simulink model "pmsm_vector_ctrl_osm_2021_07_20"  (R2020a)
settings: Solver=daessc  StartTime=0.0  StopTime=simlength  MaxStep=Ts/10
values from neighbouring files (symbols this model uses):
  dead_time = 0    [init_pmsm_2021_07_20_newDesign.m]    (also in init_pmsm_2021_07_20_oldDesign.m)
  delayINV_modA = 0    [init_pmsm_2021_07_20_newDesign.m]    (also in init_pmsm_2021_07_20_oldDesign.m)
  fPWM_INV = 8e3    (= 8000)    [init_pmsm_2021_07_20_newDesign.m]    (also in init_pmsm_2021_07_20_oldDesign.m)
  Ibez = 550    [init_pmsm_2021_07_20_newDesign.m]    (also in init_pmsm_2021_07_20_oldDesign.m)
  Jm = 1    [init_pmsm_2021_07_20_newDesign.m]    (also in init_pmsm_2021_07_20_oldDesign.m)
  ki = 18    [init_pmsm_2021_07_20_newDesign.m]    (also in init_pmsm_2021_07_20_oldDesign.m)
  kp = 2    [init_pmsm_2021_07_20_newDesign.m]    (also in init_pmsm_2021_07_20_oldDesign.m)
  Ld = 2.77e-3    (= 0.00277)    [init_pmsm_2021_07_20_newDesign.m]    (also in init_pmsm_2021_07_20_oldDesign.m = 0.00267)
  Lq = 3.77e-3    (= 0.00377)    [init_pmsm_2021_07_20_newDesign.m]    (also in init_pmsm_2021_07_20_oldDesign.m = 0.00328)
  number_poles = 8    [init_pmsm_2021_07_20_newDesign.m]    (also in init_pmsm_2021_07_20_oldDesign.m)
  psi_m = 0.5    [init_pmsm_2021_07_20_newDesign.m]    (also in init_pmsm_2021_07_20_oldDesign.m = 0.37)
  simlength = 5    [init_pmsm_2021_07_20_newDesign.m]    (also in init_pmsm_2021_07_20_oldDesign.m)
  Tc = 1e-5    (= 1e-05)    [init_pmsm_2021_07_20_newDesign.m]    (also in init_pmsm_2021_07_20_oldDesign.m)
  Ts = tPWM_INV/2    (= 3.125e-05)    [init_pmsm_2021_07_20_newDesign.m]    (also in init_pmsm_2021_07_20_oldDesign.m)
libraries: nesl_utility x25, fl_lib x23, ee_lib x6, flexshaft_lib x1, pmsm_uvw_lib x1
(part 2 of 2)

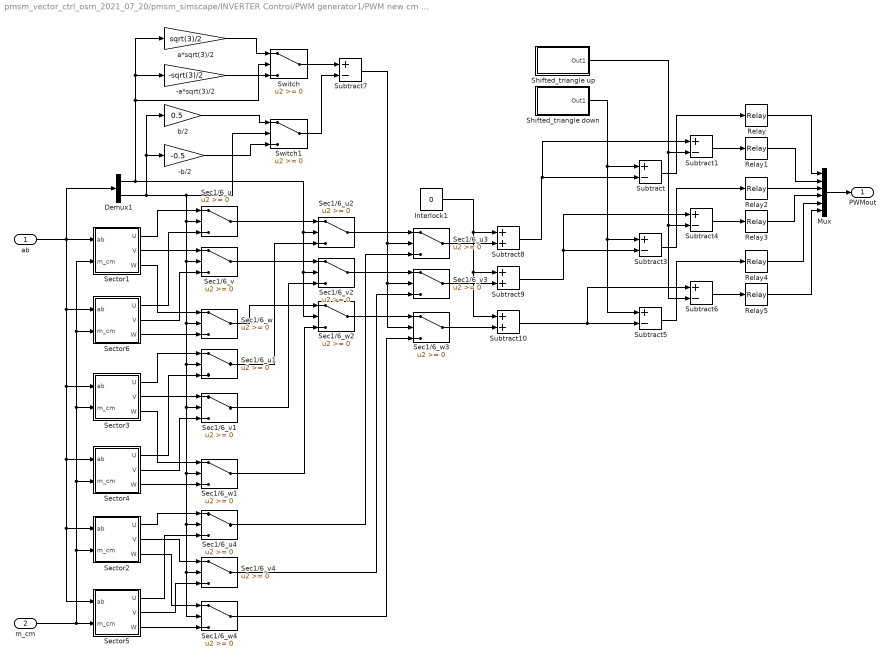
== system pmsm_vector_ctrl_osm_2021_07_20/pmsm_simscape/INVERTER Control/PWM generator1/PWM new cm modulation ==
  ab : Inport
  m_cm : Inport  Port=2
  -a*sqrt(3)/2 : Gain  Gain=-sqrt(3)/2
  -b/2 : Gain  Gain=-0.5
  Demux1 : Demux  Outputs=2
  Interlock1 : Constant  Value=0
  Mux : Mux  Inputs=6
  Relay{,1..5} (6 alike) : Relay  OnOutputValue=15
  Sec1/6_u{,1..4} (5 alike) : Switch
  Sec1/6_v{,1..4} (5 alike) : Switch
  Sec1/6_w{,1..4} (5 alike) : Switch
  Sector1 : Subsystem
  Sector2 : Subsystem
  Sector3 : Subsystem
  Sector4 : Subsystem
  Sector5 : Subsystem
  Sector6 : Subsystem
  Shifted_triangle down : Subsystem
  Shifted_triangle up : Subsystem
  Subtract{,1,3..7} (7 alike) : Sum  Inputs=+-
  Subtract10 : Sum
  Subtract8 : Sum
  Subtract9 : Sum
  Switch : Switch
  Switch1 : Switch
  a*sqrt(3)/2 : Gain  Gain=sqrt(3)/2
  b/2 : Gain  Gain=0.5
  PWMout : Outport
  wires:
  m_cm/1 -> Sector5/2(m_cm), Sector4/2(m_cm), Sector3/2(m_cm), Sector6/2(m_cm), Sector1/2(m_cm), Sector2/2(m_cm)
  Sector5/3(W) -> Sec1/6_w4/3
  Sector5/2(V) -> Sec1/6_v4/3
  Sector5/1(U) -> Sec1/6_u4/3
  Sector2/3(W) -> Sec1/6_w4/1
  Sector2/2(V) -> Sec1/6_v4/1
  Sector2/1(U) -> Sec1/6_u4/1
  Sec1/6_w4/1 -> Sec1/6_w3/3
  Sec1/6_v4/1 -> Sec1/6_v3/3
  Sec1/6_u4/1 -> Sec1/6_u3/3
  Subtract7/1 -> Sec1/6_u3/2, Sec1/6_v3/2, Sec1/6_w3/2
  Sec1/6_w2/1 -> Sec1/6_w3/1
  Sec1/6_v2/1 -> Sec1/6_v3/1
  Sec1/6_u2/1 -> Sec1/6_u3/1
  Demux1/1 -> Sec1/6_w2/2, Sec1/6_v2/2, Sec1/6_u2/2, a*sqrt(3)/2/1, -a*sqrt(3)/2/1, Switch/2
  Sector4/3(W) -> Sec1/6_w1/3
  Sector4/2(V) -> Sec1/6_v1/3
  Sector4/1(U) -> Sec1/6_u1/3
  Sector3/3(W) -> Sec1/6_w1/1
  Sector3/2(V) -> Sec1/6_v1/1
  Sector3/1(U) -> Sec1/6_u1/1
  Sec1/6_w1/1 -> Sec1/6_w2/3
  Sec1/6_v1/1 -> Sec1/6_v2/3
  Sec1/6_u1/1 -> Sec1/6_u2/3
  Sec1/6_w/1 -> Sec1/6_w2/1
  Sec1/6_v/1 -> Sec1/6_v2/1
  Sec1/6_u/1 -> Sec1/6_u2/1
  Demux1/2 -> Switch1/2, Sec1/6_w4/2, Sec1/6_v4/2, Sec1/6_u4/2, Sec1/6_w1/2, Sec1/6_v1/2, Sec1/6_u1/2, Sec1/6_w/2, Sec1/6_v/2, Sec1/6_u/2, -b/2/1, b/2/1
  Sector6/3(W) -> Sec1/6_w/3
  Sector6/2(V) -> Sec1/6_v/3
  Sector6/1(U) -> Sec1/6_u/3
  Sector1/3(W) -> Sec1/6_w/1
  Sector1/2(V) -> Sec1/6_v/1
  Sector1/1(U) -> Sec1/6_u/1
  Switch1/1 -> Subtract7/2
  Switch/1 -> Subtract7/1
  a*sqrt(3)/2/1 -> Switch/1
  -a*sqrt(3)/2/1 -> Switch/3
  -b/2/1 -> Switch1/3
  b/2/1 -> Switch1/1
  ab/1 -> Demux1/1, Sector1/1(ab), Sector6/1(ab), Sector3/1(ab), Sector4/1(ab), Sector2/1(ab), Sector5/1(ab)
  Subtract6/1 -> Relay5/1
  Subtract5/1 -> Relay4/1
  Subtract4/1 -> Relay3/1
  Subtract3/1 -> Relay2/1
  Shifted_triangle up/1(Out1) -> Subtract6/2, Subtract4/2, Subtract1/2
  Subtract1/1 -> Relay1/1
  Subtract/1 -> Relay/1
  Shifted_triangle down/1(Out1) -> Subtract5/1, Subtract3/1, Subtract/1
  Mux/1 -> PWMout/1
  Relay/1 -> Mux/1
  Relay1/1 -> Mux/2
  Relay2/1 -> Mux/3
  Relay3/1 -> Mux/4
  Relay4/1 -> Mux/5
  Relay5/1 -> Mux/6
  Sec1/6_u3/1 -> Subtract8/2
  Sec1/6_v3/1 -> Subtract9/2
  Sec1/6_w3/1 -> Subtract10/2
  Subtract10/1 -> Subtract6/1, Subtract5/2
  Subtract9/1 -> Subtract4/1, Subtract3/2
  Subtract8/1 -> Subtract1/1, Subtract/2
  Interlock1/1 -> Subtract8/1, Subtract9/1, Subtract10/1

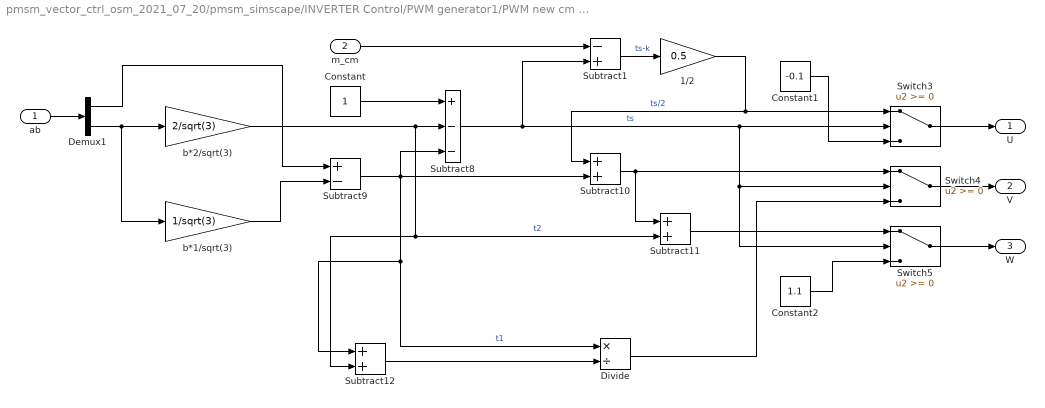
== system pmsm_vector_ctrl_osm_2021_07_20/pmsm_simscape/INVERTER Control/PWM generator1/PWM new cm modulation/Sector1 ==
  ab : Inport
  m_cm : Inport  Port=2
  1/2 : Gain  Gain=0.5
  Constant : Constant
  Constant1 : Constant  Value=-0.1
  Constant2 : Constant  Value=1.1
  Demux1 : Demux  Outputs=2
  Divide : Product  Inputs=*/
  Subtract1 : Sum  Inputs=-+
  Subtract10 : Sum
  Subtract11 : Sum
  Subtract12 : Sum
  Subtract8 : Sum  Inputs=+--
  Subtract9 : Sum  Inputs=+-
  Switch3 : Switch
  Switch4 : Switch
  Switch5 : Switch
  b*1/sqrt(3) : Gain  Gain=1/sqrt(3)
  b*2/sqrt(3) : Gain  Gain=2/sqrt(3)
  U : Outport
  V : Outport  Port=2
  W : Outport  Port=3
  wires:
  m_cm/1 -> Subtract1/1
  Switch5/1 -> W/1
  Switch4/1 -> V/1
  Switch3/1 -> U/1
  ab/1 -> Demux1/1
  Subtract8/1 -> Switch4/2, Switch5/2, Switch3/2, Subtract1/2  "ts"
  Constant/1 -> Subtract8/1
  b*2/sqrt(3)/1 -> Subtract8/2, Subtract12/2, Subtract11/2  "t2"
  Subtract9/1 -> Subtract12/1, Divide/1, Subtract10/2, Subtract8/3  "t1"
  b*1/sqrt(3)/1 -> Subtract9/2
  Subtract1/1 -> 1/2/1  "ts-k"
  Subtract10/1 -> Subtract11/1, Switch4/1
  Subtract11/1 -> Switch5/1
  Constant1/1 -> Switch3/3
  Subtract12/1 -> Divide/2
  Constant2/1 -> Switch5/3
  Divide/1 -> Switch4/3
  Demux1/1 -> Subtract9/1
  Demux1/2 -> b*2/sqrt(3)/1, b*1/sqrt(3)/1
  1/2/1 -> Switch3/1, Subtract10/1  "ts/2"

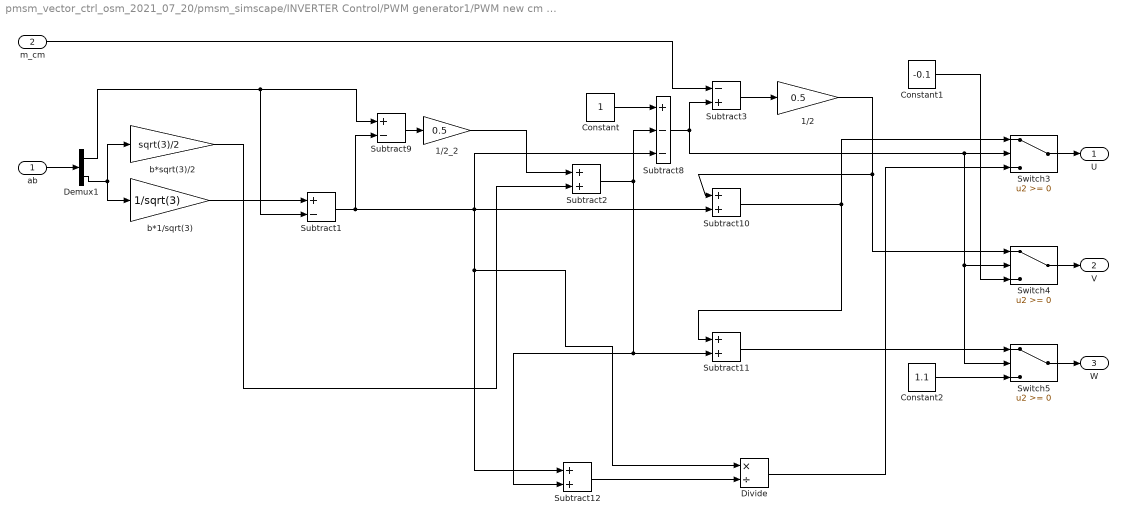
== system pmsm_vector_ctrl_osm_2021_07_20/pmsm_simscape/INVERTER Control/PWM generator1/PWM new cm modulation/Sector2 ==
  ab : Inport
  m_cm : Inport  Port=2
  1/2 : Gain  Gain=0.5
  1/2_2 : Gain  Gain=0.5
  Constant : Constant
  Constant1 : Constant  Value=-0.1
  Constant2 : Constant  Value=1.1
  Demux1 : Demux  Outputs=2
  Divide : Product  Inputs=*/
  Subtract1 : Sum  Inputs=+-
  Subtract{2,10..12} (4 alike) : Sum
  Subtract3 : Sum  Inputs=-+
  Subtract8 : Sum  Inputs=+--
  Subtract9 : Sum  Inputs=+-
  Switch3 : Switch
  Switch4 : Switch
  Switch5 : Switch
  b*1/sqrt(3) : Gain  Gain=1/sqrt(3)
  b*sqrt(3)/2 : Gain  Gain=sqrt(3)/2
  U : Outport
  V : Outport  Port=2
  W : Outport  Port=3
  wires:
  1/2/1 -> Switch4/1, Subtract10/1
  m_cm/1 -> Subtract3/1
  Subtract10/1 -> Subtract11/1, Switch3/1
  Constant2/1 -> Switch5/3
  Divide/1 -> Switch3/3
  Constant1/1 -> Switch4/3
  Subtract3/1 -> 1/2/1
  Subtract2/1 -> Subtract11/2, Subtract12/2, Subtract8/2
  b*sqrt(3)/2/1 -> Subtract2/2
  1/2_2/1 -> Subtract2/1
  Subtract9/1 -> 1/2_2/1
  Subtract1/1 -> Subtract9/2, Subtract8/3, Subtract10/2, Divide/1, Subtract12/1
  b*1/sqrt(3)/1 -> Subtract1/1
  Switch5/1 -> W/1
  Switch4/1 -> V/1
  Switch3/1 -> U/1
  ab/1 -> Demux1/1
  Subtract8/1 -> Switch5/2, Switch4/2, Switch3/2, Subtract3/2
  Constant/1 -> Subtract8/1
  Subtract11/1 -> Switch5/1
  Subtract12/1 -> Divide/2
  Demux1/1 -> Subtract1/2, Subtract9/1
  Demux1/2 -> b*sqrt(3)/2/1, b*1/sqrt(3)/1

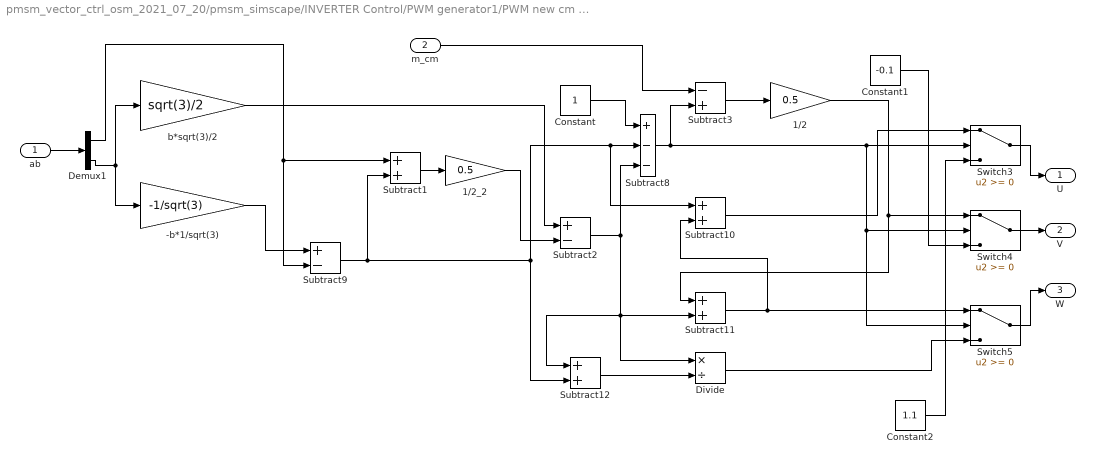
== system pmsm_vector_ctrl_osm_2021_07_20/pmsm_simscape/INVERTER Control/PWM generator1/PWM new cm modulation/Sector3 ==
  ab : Inport
  m_cm : Inport  Port=2
  -b*1/sqrt(3) : Gain  Gain=-1/sqrt(3)
  1/2 : Gain  Gain=0.5
  1/2_2 : Gain  Gain=0.5
  Constant : Constant
  Constant1 : Constant  Value=-0.1
  Constant2 : Constant  Value=1.1
  Demux1 : Demux  Outputs=2
  Divide : Product  Inputs=*/
  Subtract{1,10..12} (4 alike) : Sum
  Subtract2 : Sum  Inputs=+-
  Subtract3 : Sum  Inputs=-+
  Subtract8 : Sum  Inputs=+--
  Subtract9 : Sum  Inputs=+-
  Switch3 : Switch
  Switch4 : Switch
  Switch5 : Switch
  b*sqrt(3)/2 : Gain  Gain=sqrt(3)/2
  U : Outport
  V : Outport  Port=2
  W : Outport  Port=3
  wires:
  1/2/1 -> Switch4/1, Subtract11/1
  m_cm/1 -> Subtract3/1
  Constant1/1 -> Switch4/3
  Constant2/1 -> Switch3/3
  Divide/1 -> Switch5/3
  Subtract10/1 -> Switch3/1
  Subtract11/1 -> Subtract10/2, Switch5/1
  Subtract3/1 -> 1/2/1
  1/2_2/1 -> Subtract2/2
  Subtract1/1 -> 1/2_2/1
  b*sqrt(3)/2/1 -> Subtract2/1
  Subtract2/1 -> Subtract11/2, Divide/1, Subtract12/1, Subtract8/3
  Subtract9/1 -> Subtract12/2, Subtract8/2, Subtract10/1, Subtract1/2
  Demux1/1 -> Subtract9/2, Subtract1/1
  -b*1/sqrt(3)/1 -> Subtract9/1
  Demux1/2 -> -b*1/sqrt(3)/1, b*sqrt(3)/2/1
  Subtract12/1 -> Divide/2
  Constant/1 -> Subtract8/1
  Subtract8/1 -> Switch3/2, Switch4/2, Switch5/2, Subtract3/2
  ab/1 -> Demux1/1
  Switch3/1 -> U/1
  Switch4/1 -> V/1
  Switch5/1 -> W/1

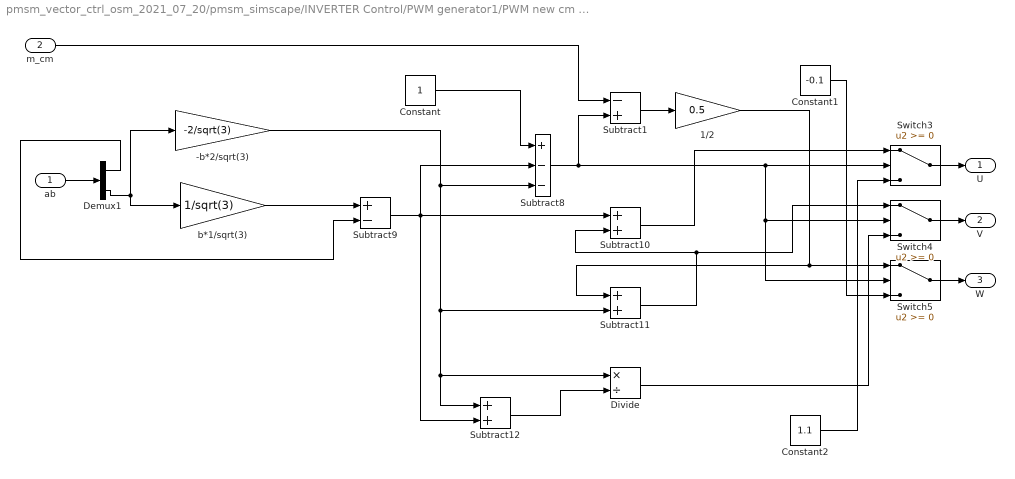
== system pmsm_vector_ctrl_osm_2021_07_20/pmsm_simscape/INVERTER Control/PWM generator1/PWM new cm modulation/Sector4 ==
  ab : Inport
  m_cm : Inport  Port=2
  -b*2/sqrt(3) : Gain  Gain=-2/sqrt(3)
  1/2 : Gain  Gain=0.5
  Constant : Constant
  Constant1 : Constant  Value=-0.1
  Constant2 : Constant  Value=1.1
  Demux1 : Demux  Outputs=2
  Divide : Product  Inputs=*/
  Subtract1 : Sum  Inputs=-+
  Subtract10 : Sum
  Subtract11 : Sum
  Subtract12 : Sum
  Subtract8 : Sum  Inputs=+--
  Subtract9 : Sum  Inputs=+-
  Switch3 : Switch
  Switch4 : Switch
  Switch5 : Switch
  b*1/sqrt(3) : Gain  Gain=1/sqrt(3)
  U : Outport
  V : Outport  Port=2
  W : Outport  Port=3
  wires:
  1/2/1 -> Switch5/1, Subtract11/1
  m_cm/1 -> Subtract1/1
  Constant1/1 -> Switch5/3
  Constant2/1 -> Switch3/3
  Divide/1 -> Switch4/3
  Subtract11/1 -> Switch4/1, Subtract10/2
  Subtract10/1 -> Switch3/1
  Subtract1/1 -> 1/2/1
  -b*2/sqrt(3)/1 -> Subtract8/3, Subtract11/2, Divide/1, Subtract12/1
  Subtract9/1 -> Subtract12/2, Subtract10/1, Subtract8/2
  Demux1/1 -> Subtract9/2
  b*1/sqrt(3)/1 -> Subtract9/1
  Switch5/1 -> W/1
  Switch4/1 -> V/1
  Switch3/1 -> U/1
  ab/1 -> Demux1/1
  Subtract8/1 -> Switch5/2, Switch4/2, Switch3/2, Subtract1/2
  Constant/1 -> Subtract8/1
  Subtract12/1 -> Divide/2
  Demux1/2 -> b*1/sqrt(3)/1, -b*2/sqrt(3)/1

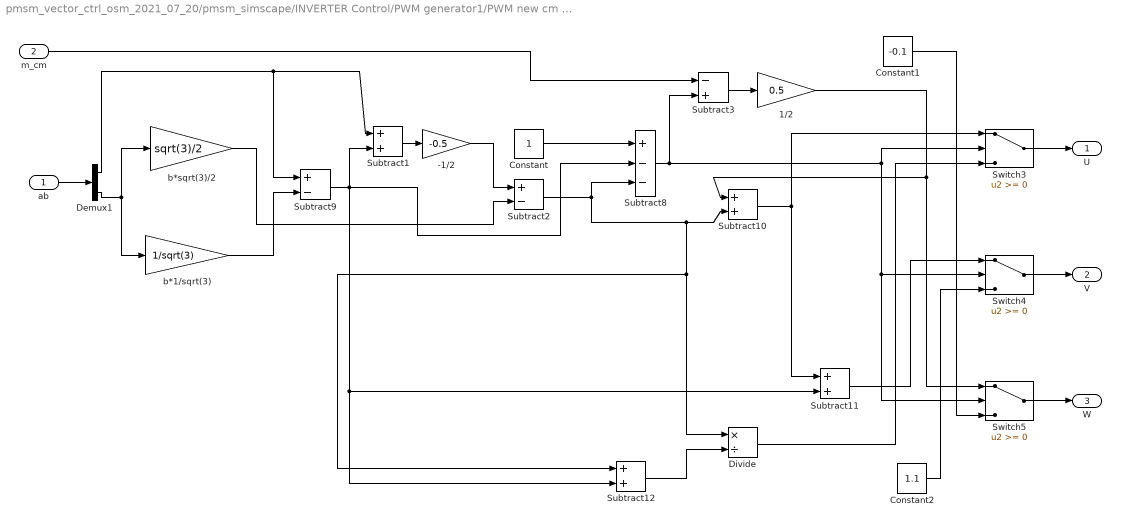
== system pmsm_vector_ctrl_osm_2021_07_20/pmsm_simscape/INVERTER Control/PWM generator1/PWM new cm modulation/Sector5 ==
  ab : Inport
  m_cm : Inport  Port=2
  -1/2 : Gain  Gain=-0.5
  1/2 : Gain  Gain=0.5
  Constant : Constant
  Constant1 : Constant  Value=-0.1
  Constant2 : Constant  Value=1.1
  Demux1 : Demux  Outputs=2
  Divide : Product  Inputs=*/
  Subtract{1,10..12} (4 alike) : Sum
  Subtract2 : Sum  Inputs=+-
  Subtract3 : Sum  Inputs=-+
  Subtract8 : Sum  Inputs=+--
  Subtract9 : Sum  Inputs=+-
  Switch3 : Switch
  Switch4 : Switch
  Switch5 : Switch
  b*1/sqrt(3) : Gain  Gain=1/sqrt(3)
  b*sqrt(3)/2 : Gain  Gain=sqrt(3)/2
  U : Outport
  V : Outport  Port=2
  W : Outport  Port=3
  wires:
  1/2/1 -> Switch5/1, Subtract10/1
  m_cm/1 -> Subtract3/1
  Constant2/1 -> Switch4/3
  Divide/1 -> Switch3/3
  Subtract11/1 -> Switch4/1
  Subtract10/1 -> Subtract11/1, Switch3/1
  Constant1/1 -> Switch5/3
  Subtract3/1 -> 1/2/1
  Subtract2/1 -> Subtract8/3, Divide/1, Subtract12/1, Subtract10/2
  b*sqrt(3)/2/1 -> Subtract2/2
  -1/2/1 -> Subtract2/1
  Subtract1/1 -> -1/2/1
  Subtract9/1 -> Subtract11/2, Subtract12/2, Subtract8/2, Subtract1/2
  Demux1/2 -> b*1/sqrt(3)/1, b*sqrt(3)/2/1
  Demux1/1 -> Subtract1/1, Subtract9/1
  Subtract12/1 -> Divide/2
  b*1/sqrt(3)/1 -> Subtract9/2
  Constant/1 -> Subtract8/1
  Subtract8/1 -> Switch3/2, Switch4/2, Switch5/2, Subtract3/2
  ab/1 -> Demux1/1
  Switch3/1 -> U/1
  Switch4/1 -> V/1
  Switch5/1 -> W/1

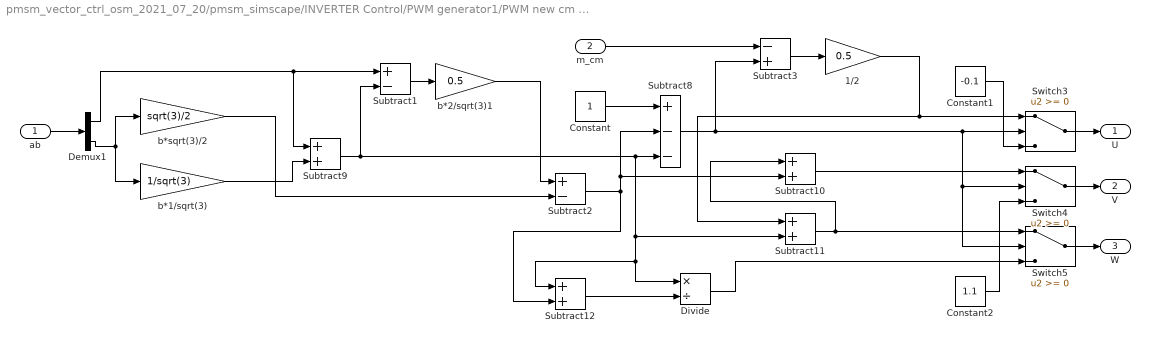
== system pmsm_vector_ctrl_osm_2021_07_20/pmsm_simscape/INVERTER Control/PWM generator1/PWM new cm modulation/Sector6 ==
  ab : Inport
  m_cm : Inport  Port=2
  1/2 : Gain  Gain=0.5
  Constant : Constant
  Constant1 : Constant  Value=-0.1
  Constant2 : Constant  Value=1.1
  Demux1 : Demux  Outputs=2
  Divide : Product  Inputs=*/
  Subtract1 : Sum  Inputs=+-
  Subtract{9..12} (4 alike) : Sum
  Subtract2 : Sum  Inputs=+-
  Subtract3 : Sum  Inputs=-+
  Subtract8 : Sum  Inputs=+--
  Switch3 : Switch
  Switch4 : Switch
  Switch5 : Switch
  b*1/sqrt(3) : Gain  Gain=1/sqrt(3)
  b*2/sqrt(3)1 : Gain  Gain=0.5
  b*sqrt(3)/2 : Gain  Gain=sqrt(3)/2
  U : Outport
  V : Outport  Port=2
  W : Outport  Port=3
  wires:
  1/2/1 -> Switch3/1, Subtract11/1
  m_cm/1 -> Subtract3/1
  Constant2/1 -> Switch4/3
  Divide/1 -> Switch5/3
  Subtract2/1 -> Subtract12/2, Subtract10/2, Subtract8/2
  b*sqrt(3)/2/1 -> Subtract2/2
  b*2/sqrt(3)1/1 -> Subtract2/1
  Subtract1/1 -> b*2/sqrt(3)1/1
  Demux1/2 -> b*1/sqrt(3)/1, b*sqrt(3)/2/1
  Demux1/1 -> Subtract1/1, Subtract9/1
  Subtract12/1 -> Divide/2
  Constant1/1 -> Switch3/3
  Subtract11/1 -> Subtract10/1, Switch5/1
  Subtract10/1 -> Switch4/1
  Subtract3/1 -> 1/2/1
  b*1/sqrt(3)/1 -> Subtract9/2
  Subtract9/1 -> Subtract8/3, Subtract11/2, Divide/1, Subtract12/1, Subtract1/2
  Constant/1 -> Subtract8/1
  Subtract8/1 -> Switch3/2, Switch4/2, Switch5/2, Subtract3/2
  ab/1 -> Demux1/1
  Switch3/1 -> U/1
  Switch4/1 -> V/1
  Switch5/1 -> W/1

== system pmsm_vector_ctrl_osm_2021_07_20/pmsm_simscape/INVERTER Control/PWM generator1/PWM new cm modulation/Shifted_triangle down ==
  Constant1 : Constant  Value=1/2-dead_time*fPWM_INV
  Gain1 : Gain  Gain=1/(pi)
  Sine Wave1 : Sin  Frequency=fPWM_INV*2*pi  Phase=-pi/2+delayINV_modA
  Subtract12 : Sum
  Trigonometric Function2 : Trigonometry  Operator=asin
  Out1 : Outport
  wires:
  Subtract12/1 -> Out1/1
  Gain1/1 -> Subtract12/1
  Constant1/1 -> Subtract12/2
  Sine Wave1/1 -> Trigonometric Function2/1
  Trigonometric Function2/1 -> Gain1/1

== system pmsm_vector_ctrl_osm_2021_07_20/pmsm_simscape/INVERTER Control/PWM generator1/PWM new cm modulation/Shifted_triangle up ==
  Constant1 : Constant  Value=1/2+dead_time*fPWM_INV
  Gain1 : Gain  Gain=1/(pi)
  Sine Wave1 : Sin  Frequency=fPWM_INV*2*pi  Phase=-pi/2+delayINV_modA
  Subtract12 : Sum
  Trigonometric Function2 : Trigonometry  Operator=asin
  Out1 : Outport
  wires:
  Trigonometric Function2/1 -> Gain1/1
  Sine Wave1/1 -> Trigonometric Function2/1
  Constant1/1 -> Subtract12/2
  Gain1/1 -> Subtract12/1
  Subtract12/1 -> Out1/1

== matlab function pmsm_vector_ctrl_osm_2021_07_20/mtpa ==
  data: Ld input; Lq input; psi_m input; iq input; id output; Ibez input
function id  = mtpa(Ld,Lq,psi_m,iq,Ibez)



id = (psi_m/2/(Lq-Ld)-sqrt(psi_m^2/4/(Lq-Ld)^2+(iq*Ibez)^2))/Ibez;
end
